simulink model "sf_multfuncout"  (R2017b)
settings: Solver=ode45  StartTime=0.0  StopTime=30  MaxStep=1  RelTol=1e-3  EnableMultiTasking=on
settings Model: FPTRunName=Active  ExtModeAutoUpdateStatusClock=off  Creator=The MathWorks, Inc.  LastModifiedBy=The MathWorks, Inc.
settings DataIOCC: LimitDataPoints=on  SaveFormat=Array
settings OptimizationCC: BooleanDataType=off  ExpressionDepthLimit=2147483647  InitFltsAndDblsToZero=on  EfficientMapNaN2IntZero=off  LifeSpan=inf
settings DebuggingCC: SaveWithParameterizedLinksMsg=none  UnderspecifiedInitializationDetection=Classic  MergeDetectMultiDrivingBlocksExec=none  SignalResolutionControl=TryResolveAllWithWarning  MultiTaskDSMMsg=warning  MultiTaskCondExecSysMsg=none  FcnCallInpInsideContextMsg=warning  StateNameClashWarn=warning  StrictBusMsg=None  SFUnexpectedBacktrackingDiag=warning  SFNoUnconditionalDefaultTransitionDiag=warning  SFExecutionAtInitializationDiag=none
settings HardwareCC: ProdBitPerPointer=32  ProdBitPerSizeT=32  ProdBitPerPtrDiffT=32  ProdLargestAtomicFloat=None  ProdIntDivRoundTo=Undefined  ProdEndianess=Unspecified  ProdWordSize=32  ProdHWDeviceType=32-bit Generic  TargetUnknown=on
settings ModelReferenceCC: PropagateSignalLabelsOutOfModel=off
settings SFSimCC: SimParseCustomCode=off
settings CodeAppCC: StateflowObjectComments=on
settings GRTTargetCC: TargetFcnLib=ansi_tfl_tmw.mat  TargetLangStandard=C89/C90 (ANSI)  GeneratePreprocessorConditionals=Disable all  CombineOutputUpdateFcns=off  GRTInterface=on
settings ConfigComp: CovMetricSettings=dcmtr  CovHtmlReporting=on  CovSaveCumulativeToWorkspaceVar=on  CovSaveSingleToWorkspaceVar=on  CovExternalEMLEnable=off  CovSFcnEnable=off

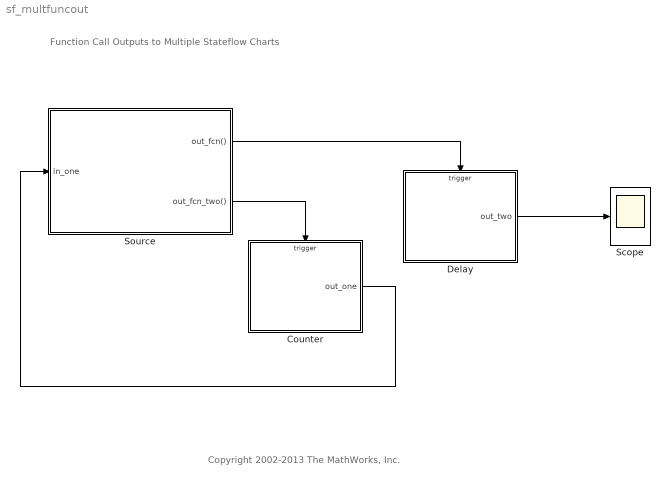
== system sf_multfuncout ==
  note: Function Call Outputs to Multiple Stateflow Charts
  note: Copyright 2002-2013 The MathWorks, Inc.
  Counter : Stateflow chart  TreatAsAtomicUnit=on
  Delay : Stateflow chart  TreatAsAtomicUnit=on
  Scope : Scope
  Source : Stateflow chart  TreatAsAtomicUnit=on
  wires:
  Source/2(out_fcn_two()) -> Counter/Trigger
  Source/1(out_fcn()) -> Delay/Trigger
  Delay/1(out_two) -> Scope/1
  Counter/1(out_one) -> Source/1(in_one)

== stateflow chart sf_multfuncout/Source ==
  state A
  state B
  state C
  (default) -> A
  A -> B : /{out_fcn_two;}
  B -> A [order 2] : /{out_fcn_two;}
  C -> A
  B -> C [order 1] : [in_one>10]/{out_fcn;}
  data: in_one input double
  events: out_fcn output FUNCTION_CALL_EVENT; out_fcn_two output FUNCTION_CALL_EVENT

== stateflow chart sf_multfuncout/Counter ==
  state A
    en:out_one=1;
    du:out_one = out_one + 1;
  (default) -> A
  data: out_one output double
  events: event input FUNCTION_CALL_EVENT

== stateflow chart sf_multfuncout/Delay ==
  state A
    en:out_two=1;
    du:out_two = out_two + 1;
  (default) -> A
  data: out_two output double
  events: event input FUNCTION_CALL_EVENT
